simulink model "qam16_ser"  (Simulink 8.3)
settings: Solver=ode45  StartTime=0.0  StopTime=1000000  RelTol=1e-3
libraries: commdigbbndam3 x2, commchan3 x1, commsink2 x1, commrandsrc2 x1
settings Model: Creator=Yang  LastModifiedBy=Yang
settings DataIOCC: SignalLoggingName=sigsOut
settings DebuggingCC: SaveWithParameterizedLinksMsg=none  SignalResolutionControl=TryResolveAllWithWarning  SolverPrmCheckMsg=none  MultiTaskDSMMsg=warning  MultiTaskCondExecSysMsg=none  StateNameClashWarn=none
settings HardwareCC: TargetUnknown=on
settings RTWCC: IncludeERTFirstTime=on

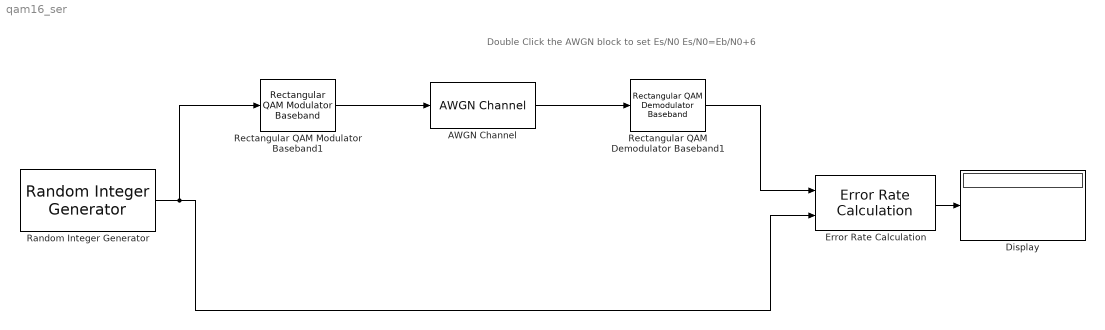
== system qam16_ser ==
  note: Double Click the AWGN block to set  Es/N0
      | Es/N0=Eb/N0+6
  AWGN Channel : commchan3/AWGN Channel  InputProcessing=Inherited (this choice will be removed - see release notes)  seed=1000  noiseMode="Signal to noise ratio  (Es/No)"  EbNodB=10  EsNodB=10+6  SNRdB=10  bitsPerSym=1  Ps=1  Tsym=1  variance=1
  Display : Display
  Error Rate Calculation : commsink2/Error Rate Calculation  N=0  st_delay=0  cp_mode=Entire frame  subframe=[]  PMode=Port  WsName=ErrorVec  RsMode2=off  stop=on  numErr=1000  maxBits=2e7
  Random Integer Generator : commrandsrc2/Random Integer Generator  mul=16  seed=5488  Ts=1  frameBased=off  sampPerFrame=1  orient=off  outDataType=double
  Rectangular QAM Demodulator Baseband1 : commdigbbndam3/Rectangular QAM Demodulator Baseband  M=16  PowType=Min. distance between symbols  MinDist=1  AvgPow=1  PeakPow=1  Ph=0  Dec=Gray  Mapping=[0:15]  OutType=Integer  DecType=Hard decision  VarSource=Dialog  Variance=1  outDtype1=Inherit via internal rule  outDtype2=Inherit via internal rule  derotateFactorWordLen=16  denormFactorWordLen=16  prodOutWordLen=32  prodOutRoundingMode=Floor  prodOutOverflowMode=Wrap  sumWordLen=32
  Rectangular QAM Modulator Baseband1 : commdigbbndam3/Rectangular QAM Modulator Baseband  M=16  InType=Integer  Enc=Gray  Mapping=[0:15]  PowType=Min. distance between symbols  MinDist=1  AvgPow=1  PeakPow=1  Ph=0  outDtype=double  outWordLen=16  outUDDataType=sfix(16)  outFracLenMode=Best precision  outFracLen=15
  wires:
  Random Integer Generator/1 -> Rectangular QAM Modulator Baseband1/1, Error Rate Calculation/2
  Rectangular QAM Demodulator Baseband1/1 -> Error Rate Calculation/1
  AWGN Channel/1 -> Rectangular QAM Demodulator Baseband1/1
  Rectangular QAM Modulator Baseband1/1 -> AWGN Channel/1
  Error Rate Calculation/1 -> Display/1
